simulink model "project_3"  (R2020a)
settings: Solver=VariableStepAuto  StartTime=0.0  StopTime=10.0  MaxStep=0.001  RelTol=1e-3
values from neighbouring files (symbols this model uses):
  b = 3.5077E-6    (= 3.5077e-06)    [project_10m.m]    (also in project_3m.m = 10; project_7m.m = 10; project_8m.m = 10; project_9m.m = 50)
  F = 2    [project2_2.m]    (also in project_3m.m = 1)
  k = 20    [project_3m.m]    (also in project_7m.m; project_8m.m)
  m = 1    [project_3m.m]    (also in project_7m.m; project_8m.m; project_9m.m = 1000)
libraries: dspsrcs4 x1
settings Model: Creator=Matt  LastModifiedBy=Matt
settings DataIOCC: ReturnWorkspaceOutputs=off

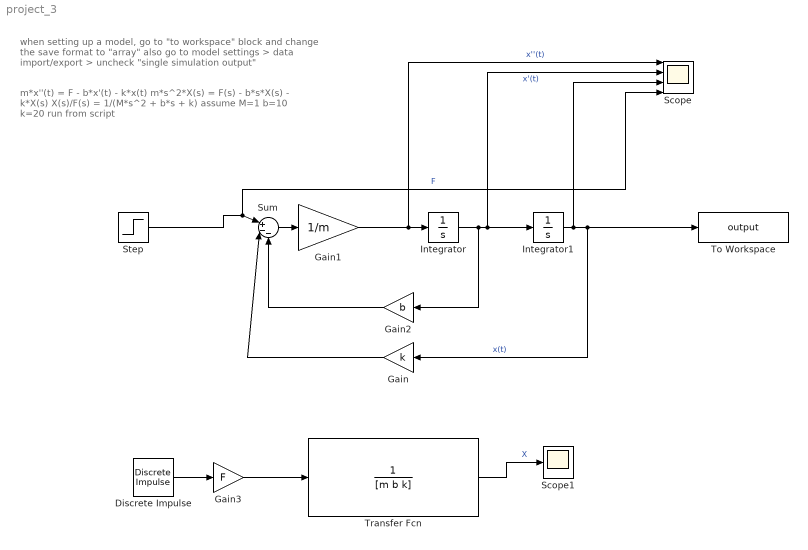
== system project_3 ==
  note: m*x''(t) = F - b*x'(t) - k*x(t)
      | m*s^2*X(s) = F(s) - b*s*X(s) - k*X(s)
      | X(s)/F(s) = 1/(M*s^2 + b*s + k)
      | assume M=1 b=10 k=20
      | run from script
  note: when setting up a model, go to "to workspace" block and change the save format to "array"
      | also go to model settings > data import/export > uncheck "single simulation output"
  Discrete Impulse : dspsrcs4/Discrete  Impulse  Delay=0  SampleTime=1  FrameSample=1  OutputFrames=off  dataType=double  isSigned=on  wordLen=16  udDataType=sfix(16)  fracBitsMode=Best precision  numFracBits=15  OutDataTypeStr=double  LastOutDataTypeStr=double
  Gain : Gain  Gain=k
  Gain1 : Gain  Gain=1/m
  Gain2 : Gain  Gain=b
  Gain3 : Gain  Gain=F
  Integrator : Integrator
  Integrator1 : Integrator
  Scope : Scope  NumInputPorts=4
  Scope1 : Scope
  Step : Step  After=F  SampleTime=0
  Sum : Sum  Inputs=|+--
  To Workspace : ToWorkspace  VariableName=output  SampleTime=-1
  Transfer Fcn : TransferFcn  Denominator=[m b k]
  wires:
  Step/1 -> Scope/4, Sum/1  "F"
  Gain/1 -> Sum/2
  Integrator/1 -> Gain2/1, Scope/2, Integrator1/1  "x'(t)"
  Sum/1 -> Gain1/1
  Gain1/1 -> Integrator/1, Scope/1  "x''(t)"
  Integrator1/1 -> Scope/3, To Workspace/1, Gain/1  "x(t)"
  Gain2/1 -> Sum/3
  Transfer Fcn/1 -> Scope1/1  "X"
  Discrete Impulse/1 -> Gain3/1
  Gain3/1 -> Transfer Fcn/1
